simulink subsystem "Sub_IR"  (R2023b)
settings: Solver=VariableStepAuto  StartTime=0.0  StopTime=10.0  RelTol=1e-3
libraries: arduinolib x2
settings Model: Creator=Usuario  LastModifiedBy=Usuario

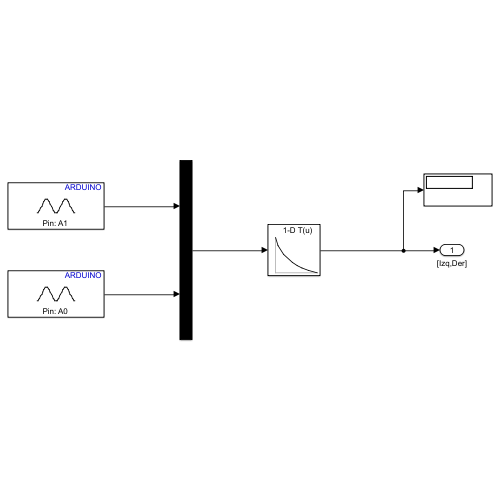
[thumbnail: Simulink's stored preview of the top-level diagram]
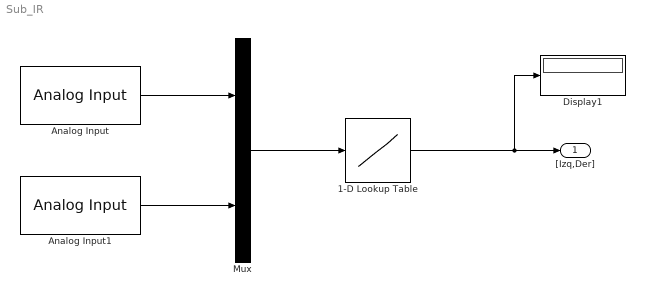
== system Sub_IR ==
  1-D Lookup Table : Lookup_n-D  NumberOfTableDimensions=1  BreakpointsForDimension1=[121;133;158;197;217;240;266;306]  BreakpointsForDimension1DataTypeStr=double  Table=[60;50;40;30;27;24;21;18]  TableDataTypeStr=double  ExtrapMethod=Clip  InternalRulePriority=Speed  OutDataTypeStr=double  RndMeth=Simplest
  Analog Input : arduinolib/Analog Input  pinNumber=1  ReadResultsOnly=off  ConversionTriggerSource=Software  ExternalTriggerType=uint32( 0 )  OutputDataType=uint16  EnableConversionCompleteNotify=off  EnableOuputStatus=off  SampleTime=-1  blockPlatform=arduino
  Analog Input1 : arduinolib/Analog Input  pinNumber=0  ReadResultsOnly=off  ConversionTriggerSource=Software  ExternalTriggerType=uint32( 0 )  OutputDataType=uint16  EnableConversionCompleteNotify=off  EnableOuputStatus=off  SampleTime=-1  blockPlatform=arduino
  Display1 : Display
  Mux : Mux  Inputs=2
  "[Izq,Der]" : Outport
  wires:
  Mux/1 -> 1-D Lookup Table/1
  Analog Input1/1 -> Mux/2
  Analog Input/1 -> Mux/1
  1-D Lookup Table/1 -> Display1/1, "[Izq,Der]"/1
